simulink model "GPC_ss"  (R2020b)
settings: Solver=VariableStepAuto  StartTime=0.0  StopTime=35  RelTol=1e-3
undefined symbols (not defined in the file): A_ss, D_ss, H_ss, KE_ss, KF_ss, Kr_ss
libraries: cstblocks x1
settings Model: Creator=LACER_GMG  LastModifiedBy=GMG

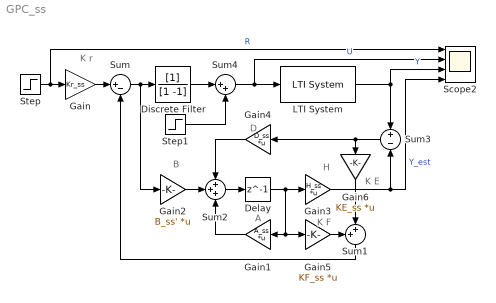
== system GPC_ss ==
  note: D
  note: A
  note: B
  note: K F
  note: K E
  note: H
  note: K r
  Delay : Delay  DelayLength=1  InitialCondition=[0 0]  SampleTime=1
  Discrete Filter : DiscreteFilter  Denominator=[1 -1]  FilterStructure=Direct form I  SampleTime=1
  Gain : Gain  Gain=Kr_ss
  Gain1 : Gain  Gain=A_ss  Multiplication=Matrix(K*u)
  Gain2 : Gain  Gain=B_ss'  Multiplication=Matrix(K*u)
  Gain3 : Gain  Gain=H_ss  Multiplication=Matrix(K*u)
  Gain4 : Gain  Gain=D_ss  Multiplication=Matrix(K*u)
  Gain5 : Gain  Gain=KF_ss  Multiplication=Matrix(K*u)
  Gain6 : Gain  Gain=KE_ss  Multiplication=Matrix(K*u)
  LTI System : cstblocks/LTI System  sys=P_ss  IC=[]
  Scope2 : Scope  NumInputPorts=4
  Step : Step  SampleTime=1
  Step1 : Step  Time=15  SampleTime=0
  Sum : Sum  Inputs=|+-
  Sum1 : Sum  Inputs=++|
  Sum2 : Sum  Inputs=+++
  Sum3 : Sum  Inputs=+|-
  Sum4 : Sum  Inputs=|++
  wires:
  Step/1 -> Scope2/1, Gain/1  "R"
  Discrete Filter/1 -> Sum4/1
  Sum1/1 -> Sum/2
  Gain2/1 -> Sum2/2
  Sum3/1 -> Gain4/1, Gain6/1
  Gain3/1 -> Sum3/2, Scope2/4  "Y_est"
  Delay/1 -> Gain3/1, Gain5/1, Gain1/1
  Gain4/1 -> Sum2/1
  Sum2/1 -> Delay/1
  Gain1/1 -> Sum2/3
  Gain5/1 -> Sum1/1
  Gain6/1 -> Sum1/2
  Gain/1 -> Sum/1
  Sum/1 -> Gain2/1, Discrete Filter/1
  LTI System/1 -> Scope2/3, Sum3/1  "Y"
  Sum4/1 -> Scope2/2, LTI System/1  "U"
  Step1/1 -> Sum4/2
